simulink model "SMD_MSR_Sim_V1"  (R2019a)
settings: Solver=ode45  StartTime=0.0  StopTime=simtime  MaxStep=ts_max
values from neighbouring files (symbols this model uses):
  a_f = 1E-5*depl_fuel_temp_coef(depl_index)    [MSDR_parameters_V5.m]    (also in SMD_MSR_Para_V1.m)
  a_g = 1E-5*depl_grap_temp_coef(depl_index)    [MSDR_parameters_V5.m]    (also in SMD_MSR_Para_V1.m)
  beta = depl_beta(depl_index,:)    [MSDR_parameters_V5.m]    (also in SMD_MSR_Para_V1.m)
  beta_t = sum(beta)    [MSDR_parameters_V5.m]    (also in SMD_MSR_Para_V1.m)
  Block_UHE = 200000    [step_insertion_depl.m]
  DHRS_Power = P*(0.10)    (= 0.8)    [step_insertion_depl.m]
  DHRS_time = 200000    [step_insertion_depl.m]
  DHRS_TIME_K = 10    [MSDR_parameters_V5.m]    (also in SMD_MSR_Para_V1.m)
  Epsilon = 1E-3    (= 0.001)    [MSDR_parameters_V5.m]    (also in SMD_MSR_Para_V1.m)
  Fiss_factor = 2.464783802008740e-03    (= 0.00246478380201)    [MSDR_parameters_V5.m]    (also in SMD_MSR_Para_V1.m)
  gamma0 = 9.635981959409105e-01    (= 0.963598195941)    [MSDR_parameters_V5.m]    (also in SMD_MSR_Para_V1.m)
  gamma1 = 3.560674858154914e-02    (= 0.0356067485815)    [MSDR_parameters_V5.m]    (also in SMD_MSR_Para_V1.m)
  gamma2 = 7.950554775404400e-04    (= 0.00079505547754)    [MSDR_parameters_V5.m]    (also in SMD_MSR_Para_V1.m)
  gamma_I = 5.1135e-2    (= 0.051135)    [MSDR_parameters_V5.m]    (also in SMD_MSR_Para_V1.m)
  gamma_Xe = 1.1628e-2    (= 0.011628)    [MSDR_parameters_V5.m]    (also in SMD_MSR_Para_V1.m)
  hA_fg = [h_fg*A_fg/2, h_fg*A_fg/2]    [MSDR_parameters_V5.m]    (also in SMD_MSR_Para_V1.m = Psf_li*(0.02*9/5)/nn_f)
  hA_pn = (Psf_li*ha_p)/nn_s    [SMD_MSR_Para_V1.m]
  hA_rpn = (Psf_li*h_roverall*A_rad)/nn_rs    [SMD_MSR_Para_V1.m]
  hA_rsn = (Psf_li*h_roverall*A_rad)/nn_rs    [SMD_MSR_Para_V1.m]
  hA_sn = (Psf_li*ha_s)/nn_s    [SMD_MSR_Para_V1.m]
  I_0 = gamma_I*Sig_f_msdr*phi_0/lam_I    [MSDR_parameters_V5.m]    (also in SMD_MSR_Para_V1.m)
  k_1 = 0.5    [SMD_MSR_Para_V1.m]
  k_2 = 0.5    [SMD_MSR_Para_V1.m]
  k_f1 = k_f/nn_f    (= 0.465)    [SMD_MSR_Para_V1.m]
  k_f2 = k_f/nn_f    (= 0.465)    [SMD_MSR_Para_V1.m]
  k_g = 0.07    [SMD_MSR_Para_V1.m]
  K_pump = 1/5    (= 0.2)    [MSDR_parameters_V5.m]    (also in SMD_MSR_Para_V1.m = 10000000)
  Lam = depl_Lam(depl_index)    [MSDR_parameters_V5.m]    (also in SMD_MSR_Para_V1.m)
  lam = [0.0124, 0.0305, 0.111, 0.301, 1.14, 3.01]    [MSDR_parameters_V5.m]    (also in SMD_MSR_Para_V1.m = [1.240E-02, 3.05E-02, 1.11E-01, 3.01E-01, 1.140E+00, 3.014E+)
  lam_bubl = 2.0e-2    (= 0.02)    [MSDR_parameters_V5.m]    (also in SMD_MSR_Para_V1.m)
  lam_I = 2.875e-5    (= 2.875e-05)    [MSDR_parameters_V5.m]    (also in SMD_MSR_Para_V1.m)
  lam_Xe = 2.0916e-5    (= 2.0916e-05)    [MSDR_parameters_V5.m]    (also in SMD_MSR_Para_V1.m)
  lambda0 = 0.0945298    [MSDR_parameters_V5.m]    (also in SMD_MSR_Para_V1.m)
  lambda1 = 0.00441957    [MSDR_parameters_V5.m]    (also in SMD_MSR_Para_V1.m)
  lambda2 = 8.60979e-05    [MSDR_parameters_V5.m]    (also in SMD_MSR_Para_V1.m)
  m_f_t = total_mp_phx + core_fm    [MSDR_parameters_V5.m]    (also in SMD_MSR_Para_V1.m = W_f*(tau_l+tau_c))
  mcp_f1 = mn_f*scp_f    [SMD_MSR_Para_V1.m]
  mcp_f2 = mn_f*scp_f    [SMD_MSR_Para_V1.m]
  mcp_g1 = m_g*scp_g    [SMD_MSR_Para_V1.m]
  mcp_pn = mn_p*cp_p    [SMD_MSR_Para_V1.m]
  mcp_rpn = mn_rp*cp_rp    [SMD_MSR_Para_V1.m]
  mcp_rsn = mn_rs*scp_rs    [SMD_MSR_Para_V1.m]
  mcp_sn = mn_s*scp_s    [SMD_MSR_Para_V1.m]
  mcp_tn = m_tn*scp_t    [SMD_MSR_Para_V1.m]
  mn_f = (m_f/nn_f)    [SMD_MSR_Para_V1.m]
  mn_p = m_p/nn_p    [SMD_MSR_Para_V1.m]
  mn_pi_c_hx = W_f*tau_c_hx    (= 1783.7391)    [MSDR_parameters_V5.m]    (also in SMD_MSR_Para_V1.m = (W_f*tau_c_hx))
  mn_pi_hx_c = W_f*3*tau_hx_c + m_fm    (= 15330.1773)    [MSDR_parameters_V5.m]    (also in SMD_MSR_Para_V1.m = (W_f*tau_hx_c))
  mn_piDHRS = W_f*(0.1)    (= 498.948)    [MSDR_parameters_V5.m]    (also in SMD_MSR_Para_V1.m = (W_f*tau_DHRS))
  mn_piFP = (W_f*tau_FP)    [SMD_MSR_Para_V1.m]
  mn_rp = m_rp/nn_rp    [SMD_MSR_Para_V1.m]
  mn_rs = m_rs/nn_rs    [SMD_MSR_Para_V1.m]
  mn_s = m_s/nn_s    [SMD_MSR_Para_V1.m]
  n_frac0 = 1    [SMD_MSR_Para_V1.m]
  omega = 10.00000    (= 10)    [step_insertion_depl.m]
  P = 8    [step_insertion_depl.m]
  phi_0 = P/(3.04414e-17*1e6*Sig_f_msdr)    [MSDR_parameters_V5.m]    (also in SMD_MSR_Para_V1.m)
  Power_Bleed = P*(0.00)    [MSDR_parameters_V5.m]    (also in step_insertion_depl.m = 0)
  rho_f = 751.042    [MSDR_parameters_V5.m]    (also in SMD_MSR_Para_V1.m = 2146.47)
  rho_s = 1/vss    [MSDR_parameters_V5.m]    (also in SMD_MSR_Para_V1.m = 1922)
  rhoXe_0 = (-sig_Xe/Sig_a)*(gamma_I+gamma_Xe)*Sig_f_msdr*phi_0/(lam_Xe + sig_Xe*phi_0 + lam_bubl)    [MSDR_parameters_V5.m]    (also in SMD_MSR_Para_V1.m)
  rm_power = W_f*scp_f*deltaTf_DHRS    [SMD_MSR_Para_V1.m]
  scp_f = 1.9665E-3    (= 0.0019665)    [SMD_MSR_Para_V1.m]
  scp_s = 2.39E-3    (= 0.00239)    [SMD_MSR_Para_V1.m]
  Sig_f_msdr = U_den*U_sig    [MSDR_parameters_V5.m]    (also in SMD_MSR_Para_V1.m = 0.058501076601)
  sig_Xe = 2.66449e-18    [MSDR_parameters_V5.m]    (also in SMD_MSR_Para_V1.m)
  sin_mag = 0    [step_insertion_depl.m]
  slug_time = 8.46    [step_insertion_depl.m]
  T0_f1 = Tf_in + (T0_f2-Tf_in)/2    (= 644.745)    [SMD_MSR_Para_V1.m]
  T0_f2 = 6.5727E+02    (= 657.27)    [SMD_MSR_Para_V1.m]
  T0_g1 = T0_f1+(k_g*P_MSRE/hA_fg)    [SMD_MSR_Para_V1.m]
  T0_p1 = Tp_in - (Tp_in-T0_p4)/4    (= 651.0075)    [SMD_MSR_Para_V1.m]
  T0_p2 = Tp_in - 2*(Tp_in-T0_p4)/4    (= 644.745)    [SMD_MSR_Para_V1.m]
  T0_p3 = Tp_in - 3*(Tp_in-T0_p4)/4    (= 638.4825)    [SMD_MSR_Para_V1.m]
  T0_p4 = Tf_in    (= 632.22)    [SMD_MSR_Para_V1.m]
  T0_rp = Ts_in    (= 546.11)    [SMD_MSR_Para_V1.m]
  T0_rs = 148.9    [SMD_MSR_Para_V1.m]
  T0_s1 = Ts_in + (T0_s4-Ts_in)/nn_s    (= 554.43)    [SMD_MSR_Para_V1.m]
  T0_s2 = Ts_in + 2*(T0_s4-Ts_in)/nn_s    (= 562.75)    [SMD_MSR_Para_V1.m]
  T0_s3 = Ts_in + 3*(T0_s4-Ts_in)/nn_s    (= 571.07)    [SMD_MSR_Para_V1.m]
  T0_s4 = 5.7939E+02    (= 579.39)    [SMD_MSR_Para_V1.m]
  T0_t1 = 6.253671698113207E+02    (= 625.367169811)    [SMD_MSR_Para_V1.m]
  T0_t2 = 6.115222641509436e+02    (= 611.522264151)    [SMD_MSR_Para_V1.m]
  tau_c = core_fm/W_f    [MSDR_parameters_V5.m]    (also in SMD_MSR_Para_V1.m = 8.46)
  tau_c_DHRS = (tau_c_hx - tau_DHRS)/2    (= 1.385)    [SMD_MSR_Para_V1.m]
  tau_DHRS_hx = (tau_c_hx - tau_DHRS)/2    (= 1.385)    [SMD_MSR_Para_V1.m]
  tau_FP_c = (tau_hx_c - tau_FP)/2    (= 3.835)    [SMD_MSR_Para_V1.m]
  tau_hx_FP = (tau_hx_c - tau_FP)/2    (= 3.835)    [SMD_MSR_Para_V1.m]
  tau_hx_r = 4.71    [SMD_MSR_Para_V1.m]
  tau_l = pipe_fm/W_f    [MSDR_parameters_V5.m]    (also in SMD_MSR_Para_V1.m = 16.73)
  tau_r_hx = 8.24    [SMD_MSR_Para_V1.m]
  Trip_P_pump = 20000000    [step_insertion_depl.m]
  Trip_S_pump = 20000000    [step_insertion_depl.m]
  Trs_in = 37.78    [SMD_MSR_Para_V1.m]
  vdot_f = Psf_li*7.5708E-02    [SMD_MSR_Para_V1.m]
  vdot_f_fc_pc = 0.05    [MSDR_parameters_V5.m]    (also in SMD_MSR_Para_V1.m)
  vdot_s = Psf_li*5.36265E-02    [SMD_MSR_Para_V1.m]
  W_f = 4989.48    [MSDR_parameters_V5.m]    (also in SMD_MSR_Para_V1.m = vdot_f*rho_f)
  W_p = W_f    [SMD_MSR_Para_V1.m]
  W_rp = W_s    [SMD_MSR_Para_V1.m]
  W_rs = vdot_rs*rho_rs    [SMD_MSR_Para_V1.m]
  W_s = vdot_s*rho_s    [SMD_MSR_Para_V1.m]
  Xe_0 = (gamma_Xe*Sig_f_msdr*phi_0 + lam_I*I_0)/(lam_Xe + sig_Xe*phi_0 + lam_bubl)    [MSDR_parameters_V5.m]    (also in SMD_MSR_Para_V1.m)
  Xe_og = lam_bubl*Xe_0/(lam_Xe)    [MSDR_parameters_V5.m]    (also in SMD_MSR_Para_V1.m)
undefined symbols (not defined in the file or in its folder): C0, ln
settings Model: Creator=visura96  LastModifiedBy=visura
settings SolverCC: AlgebraicLoopSolver=LineSearch
settings DataIOCC: ReturnWorkspaceOutputs=off

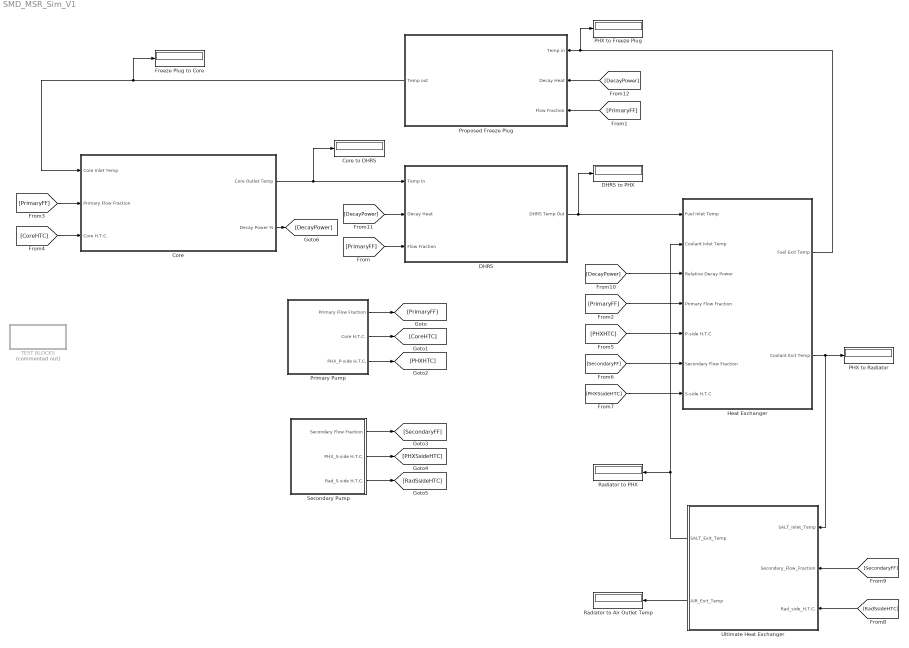
== system SMD_MSR_Sim_V1 ==
  " Heat Exchanger" : Subsystem
  Core : Subsystem
  Core to DHRS : Display
  "DHRS " : Subsystem
  DHRS to PHX : Display
  Freeze Plug to Core : Display
  PHX to Freeze Plug : Display
  PHX to Radiator : Display
  Primary Pump : Subsystem
  Proposed Freeze Plug : Subsystem
  Radiator to Air Outlet Temp : Display
  Radiator to PHX : Display
  Secondary Pump : Subsystem
  TEST BLOCKS : Subsystem  Commented=on
  Ultimate Heat Exchanger : Subsystem  Variant=on
  wires:
  Primary Pump/1(Primary Flow Fraction) -> [PrimaryFF]
  [PrimaryFF] -> Proposed Freeze Plug/3(Flow Fraction)
  [PrimaryFF] -> " Heat Exchanger"/4(Primary Flow Fraction)
  [PrimaryFF] -> Core/2(Primary Flow Fraction)
  Primary Pump/2(Core H.T.C.) -> [CoreHTC]
  [CoreHTC] -> Core/3(Core H.T.C.)
  Primary Pump/3(PHX_P-side H.T.C.) -> [PHXHTC]
  [PHXHTC] -> " Heat Exchanger"/5(P-side H.T.C)
  Secondary Pump/1(Secondary Flow Fraction) -> [SecondaryFF]
  Secondary Pump/2(PHX_S-side H.T.C.) -> [PHXSsideHTC]
  Secondary Pump/3(Rad_S-side H.T.C.) -> [RadSsideHTC]
  [SecondaryFF] -> " Heat Exchanger"/6(Secondary Flow Fraction)
  [PHXSsideHTC] -> " Heat Exchanger"/7(S-side H.T.C)
  [DecayPower] -> " Heat Exchanger"/3(Relative Decay Power)
  [DecayPower] -> Proposed Freeze Plug/2(Decay Heat)
  Core/1(Core Outlet Temp) -> Core to DHRS/1, "DHRS "/1("Temp In ")
  Core/2(Decay Power %) -> [DecayPower]
  [DecayPower] -> "DHRS "/2(Decay Heat)
  [PrimaryFF] -> "DHRS "/3(Flow Fraction)
  Proposed Freeze Plug/1(Temp out) -> Freeze Plug to Core/1, Core/1("Core Inlet Temp ")
  " Heat Exchanger"/2(Coolant Exit Temp) -> Ultimate Heat Exchanger/1(SALT_Inlet_Temp), PHX to Radiator/1
  "DHRS "/1("DHRS Temp Out ") -> " Heat Exchanger"/1(Fuel Inlet Temp), DHRS to PHX/1
  " Heat Exchanger"/1(Fuel Exit Temp) -> PHX to Freeze Plug/1, Proposed Freeze Plug/1("Temp in ")
  [RadSsideHTC] -> Ultimate Heat Exchanger/3(Rad_side_H.T.C.)
  [SecondaryFF] -> Ultimate Heat Exchanger/2(Secondary_Flow_Fraction)
  Ultimate Heat Exchanger/1(SALT_Exit_Temp) -> Radiator to PHX/1, " Heat Exchanger"/2(Coolant Inlet Temp)
  Ultimate Heat Exchanger/2(AIR_Exit_Temp) -> Radiator to Air Outlet Temp/1

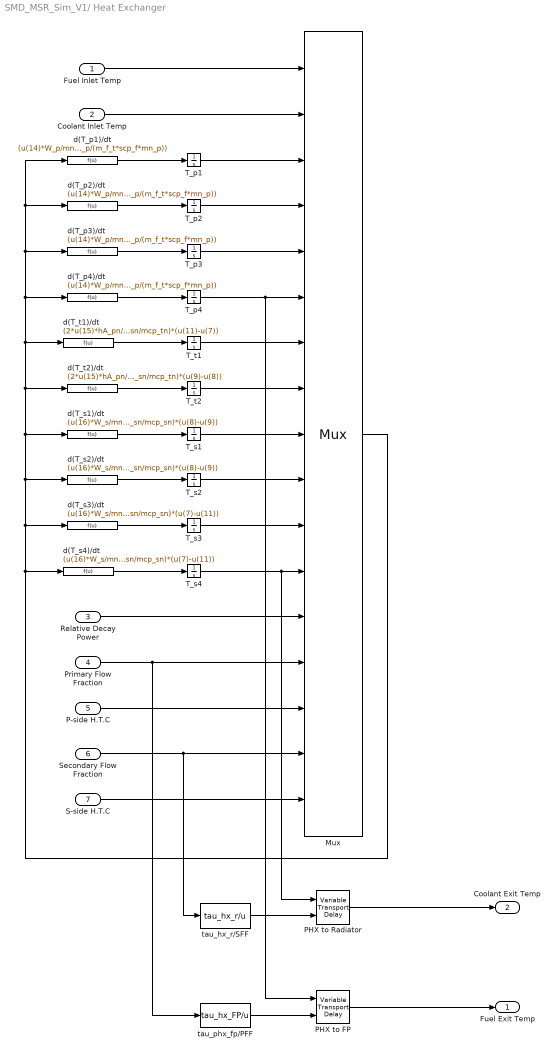
== system SMD_MSR_Sim_V1/ Heat Exchanger ==
  Fuel Inlet Temp : Inport
  Coolant Inlet Temp : Inport  Port=2
  Relative Decay Power : Inport  Port=3
  Primary Flow Fraction : Inport  Port=4
  P-side H.T.C : Inport  Port=5
  Secondary Flow Fraction : Inport  Port=6
  S-side H.T.C : Inport  Port=7
  Mux : Mux  Inputs=17
      settings: DisplayOption=signals
  PHX to FP : VariableTransportDelay  MaximumDelay=10000000000  InitialOutput=T0_p4
  PHX to Radiator : VariableTransportDelay  MaximumDelay=10000000000  InitialOutput=T0_s4
  T_p1 : Integrator  InitialCondition=T0_p1
  T_p2 : Integrator  InitialCondition=T0_p2
  "T_p3 " : Integrator  InitialCondition=T0_p3
  T_p4 : Integrator  InitialCondition=T0_p4
  T_s1 : Integrator  InitialCondition=T0_s1
  T_s2 : Integrator  InitialCondition=T0_s2
  T_s3 : Integrator  InitialCondition=T0_s3
  T_s4 : Integrator  InitialCondition=T0_s4
  T_t1 : Integrator  InitialCondition=T0_t1
  T_t2 : Integrator  InitialCondition=T0_t2
  d(T_p1)/dt : Fcn  Expr=(u(14)*W_p/mn_p)*(u(1)-u(3)) + (u(15)*hA_pn/mcp_pn)*(u(7)-u(3)) + (u(13)*P*mn_p/(m_f_t*scp_f*mn_p))
  d(T_p2)/dt : Fcn  Expr=(u(14)*W_p/mn_p)*(u(3)-u(4)) + (u(15)*hA_pn/mcp_pn)*(u(7)-u(3)) + (u(13)*P*mn_p/(m_f_t*scp_f*mn_p))
  d(T_p3)/dt : Fcn  Expr=(u(14)*W_p/mn_p)*(u(4)-u(5)) + (u(15)*hA_pn/mcp_pn)*(u(8)-u(5)) + (u(13)*P*mn_p/(m_f_t*scp_f*mn_p))
  d(T_p4)/dt : Fcn  Expr=(u(14)*W_p/mn_p)*(u(5)-u(6)) + (u(15)*hA_pn/mcp_pn)*(u(8)-u(5)) + (u(13)*P*mn_p/(m_f_t*scp_f*mn_p))
  d(T_s1)/dt : Fcn  Expr=(u(16)*W_s/mn_s)*(u(2)-u(9)) + (u(17)*hA_sn/mcp_sn)*(u(8)-u(9))
  d(T_s2)/dt : Fcn  Expr=(u(16)*W_s/mn_s)*(u(9)-u(10)) + (u(17)*hA_sn/mcp_sn)*(u(8)-u(9))
  d(T_s3)/dt : Fcn  Expr=(u(16)*W_s/mn_s)*(u(10)-u(11)) + (u(17)*hA_sn/mcp_sn)*(u(7)-u(11))
  d(T_s4)/dt : Fcn  Expr=(u(16)*W_s/mn_s)*(u(11)-u(12)) + (u(17)*hA_sn/mcp_sn)*(u(7)-u(11))
  d(T_t1)/dt : Fcn  Expr=(2*u(15)*hA_pn/mcp_tn)*(u(3)-u(7)) + (2*u(17)*hA_sn/mcp_tn)*(u(11)-u(7))
  d(T_t2)/dt : Fcn  Expr=(2*u(15)*hA_pn/mcp_tn)*(u(5)-u(8)) + (2*u(17)*hA_sn/mcp_tn)*(u(9)-u(8))
  tau_hx_r/SFF : Fcn  Expr=tau_hx_r/u
  tau_phx_fp/PFF : Fcn  Expr=tau_hx_FP/u
  Fuel Exit Temp : Outport
  Coolant Exit Temp : Outport  Port=2
  wires:
  Fuel Inlet Temp/1 -> Mux/1
  Coolant Inlet Temp/1 -> Mux/2
  d(T_p1)/dt/1 -> T_p1/1
  d(T_p2)/dt/1 -> T_p2/1
  d(T_p3)/dt/1 -> "T_p3 "/1
  d(T_p4)/dt/1 -> T_p4/1
  d(T_t1)/dt/1 -> T_t1/1
  d(T_t2)/dt/1 -> T_t2/1
  d(T_s1)/dt/1 -> T_s1/1
  d(T_s2)/dt/1 -> T_s2/1
  T_p2/1 -> Mux/4
  T_p1/1 -> Mux/3
  d(T_s3)/dt/1 -> T_s3/1
  d(T_s4)/dt/1 -> T_s4/1
  Mux/1 -> d(T_s4)/dt/1, d(T_s3)/dt/1, d(T_s2)/dt/1, d(T_s1)/dt/1, d(T_t2)/dt/1, d(T_t1)/dt/1, d(T_p4)/dt/1, d(T_p3)/dt/1, d(T_p2)/dt/1, d(T_p1)/dt/1
  "T_p3 "/1 -> Mux/5
  T_p4/1 -> PHX to FP/1, Mux/6
  T_t1/1 -> Mux/7
  T_s4/1 -> PHX to Radiator/1, Mux/12
  T_s3/1 -> Mux/11
  T_s2/1 -> Mux/10
  T_t2/1 -> Mux/8
  Relative Decay Power/1 -> Mux/13
  Primary Flow Fraction/1 -> tau_phx_fp/PFF/1, Mux/14
  P-side H.T.C/1 -> Mux/15
  Secondary Flow Fraction/1 -> tau_hx_r/SFF/1, Mux/16
  S-side H.T.C/1 -> Mux/17
  tau_hx_r/SFF/1 -> PHX to Radiator/2
  PHX to Radiator/1 -> Coolant Exit Temp/1
  T_s1/1 -> Mux/9
  PHX to FP/1 -> Fuel Exit Temp/1
  tau_phx_fp/PFF/1 -> PHX to FP/2

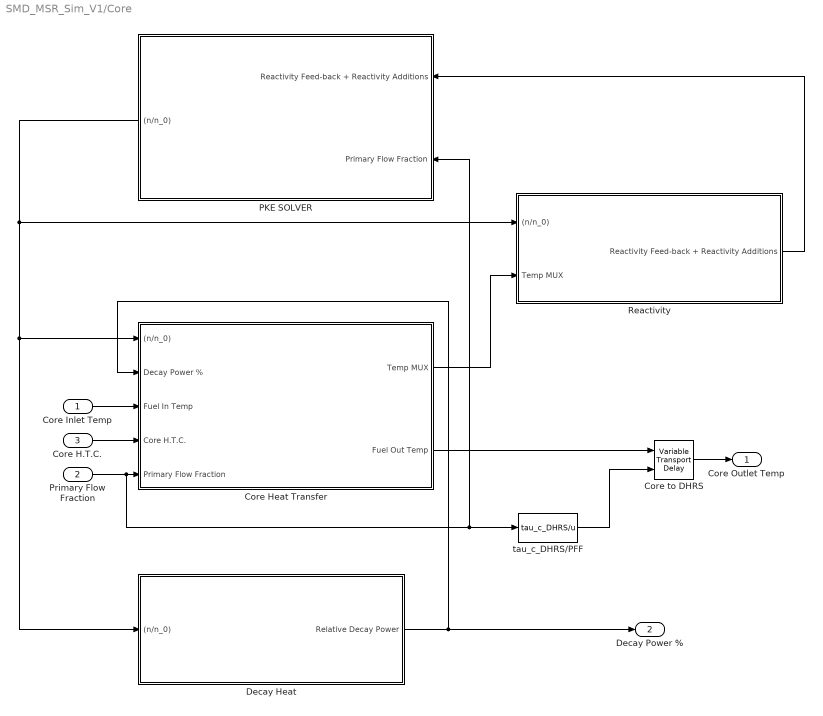
== system SMD_MSR_Sim_V1/Core ==
  "Core Inlet Temp " : Inport
  Primary Flow Fraction : Inport  Port=2
  Core H.T.C. : Inport  Port=3
  Core Heat Transfer : Subsystem
  Core to DHRS : VariableTransportDelay  MaximumDelay=10000000000  InitialOutput=T0_f2
  Decay Heat : Subsystem
  PKE SOLVER : Subsystem
  "Reactivity " : Subsystem
  tau_c_DHRS/PFF : Fcn  Expr=tau_c_DHRS/u
  Core Outlet Temp : Outport
  Decay Power % : Outport  Port=2
  wires:
  "Core Inlet Temp "/1 -> Core Heat Transfer/3(Fuel In Temp)
  Primary Flow Fraction/1 -> tau_c_DHRS/PFF/1, PKE SOLVER/2(Primary Flow Fraction), Core Heat Transfer/5(Primary Flow Fraction)
  Core H.T.C./1 -> Core Heat Transfer/4(Core H.T.C.)
  Core Heat Transfer/1(Temp MUX) -> "Reactivity "/2(Temp MUX)
  Decay Heat/1("Relative Decay Power ") -> Core Heat Transfer/2(Decay Power %), Decay Power %/1
  "Reactivity "/1(Reactivity Feed-back + Reactivity Additions) -> PKE SOLVER/1(Reactivity Feed-back + Reactivity Additions)
  PKE SOLVER/1((n/n_0)) -> Core Heat Transfer/1("(n/n_0) "), Decay Heat/1((n/n_0)), "Reactivity "/1((n/n_0))
  Core Heat Transfer/2(Fuel Out Temp) -> Core to DHRS/1
  Core to DHRS/1 -> Core Outlet Temp/1
  tau_c_DHRS/PFF/1 -> Core to DHRS/2

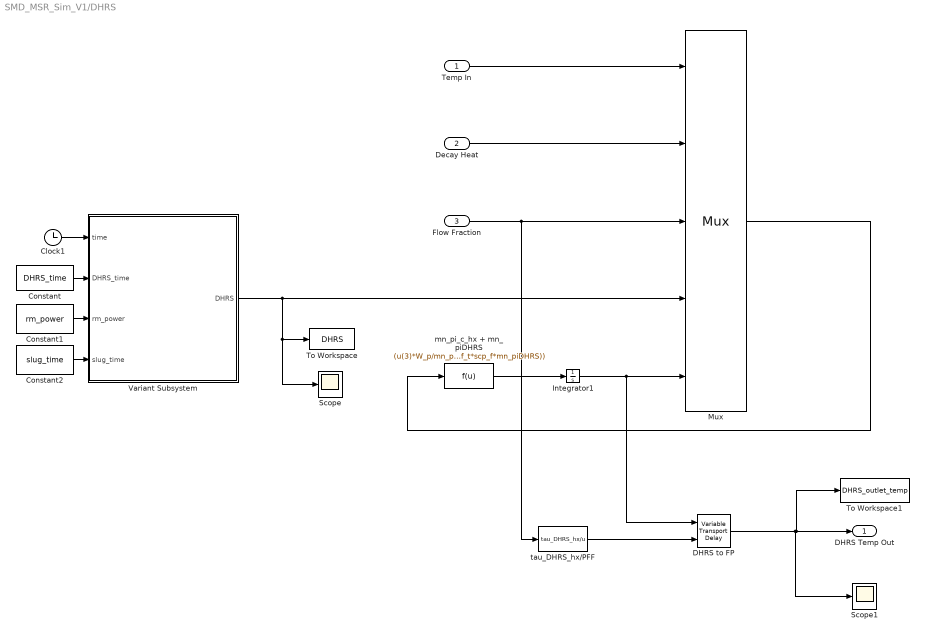
== system SMD_MSR_Sim_V1/DHRS  ==
  "Temp In " : Inport
  Decay Heat : Inport  Port=2
  Flow Fraction : Inport  Port=3
  Clock1 : Clock
  Constant : Constant  Value=DHRS_time
  Constant1 : Constant  Value=rm_power
  Constant2 : Constant  Value=slug_time
  DHRS to FP : VariableTransportDelay  MaximumDelay=10000000000  InitialOutput=T0_p1
  Integrator1 : Integrator  InitialCondition=T0_p1
  Mux : Mux  Inputs=5
      settings: DisplayOption=signals
  Scope : Scope
  Scope1 : Scope
  To Workspace : ToWorkspace  VariableName=DHRS  SaveFormat=Timeseries  SampleTime=-1
  To Workspace1 : ToWorkspace  VariableName=DHRS_outlet_temp  SampleTime=-1
  Variant Subsystem : Subsystem  Variant=on
  mn_pi_c_hx + mn_piDHRS : Fcn  Expr="(u(3)*W_p/mn_piDHRS)*(u(1) - u(5)) - (u(4)/(mn_piDHRS*scp_f))  + (u(2)*P*mn_pi_c_hx/(m_f_t*scp_f*mn_piDHRS))"
  tau_DHRS_hx/PFF : Fcn  Expr=tau_DHRS_hx/u
  "DHRS Temp Out " : Outport
  wires:
  Mux/1 -> mn_pi_c_hx + mn_piDHRS/1
  Flow Fraction/1 -> Mux/3, tau_DHRS_hx/PFF/1
  mn_pi_c_hx + mn_piDHRS/1 -> Integrator1/1
  DHRS to FP/1 -> Scope1/1, To Workspace1/1, "DHRS Temp Out "/1
  tau_DHRS_hx/PFF/1 -> DHRS to FP/2
  Integrator1/1 -> Mux/5, DHRS to FP/1
  Variant Subsystem/1(DHRS) -> To Workspace/1, Scope/1, Mux/4
  Clock1/1 -> Variant Subsystem/1(time)
  Constant/1 -> Variant Subsystem/2(DHRS_time)
  Constant1/1 -> Variant Subsystem/3(rm_power)
  Constant2/1 -> Variant Subsystem/4(slug_time)
  "Temp In "/1 -> Mux/1
  Decay Heat/1 -> Mux/2

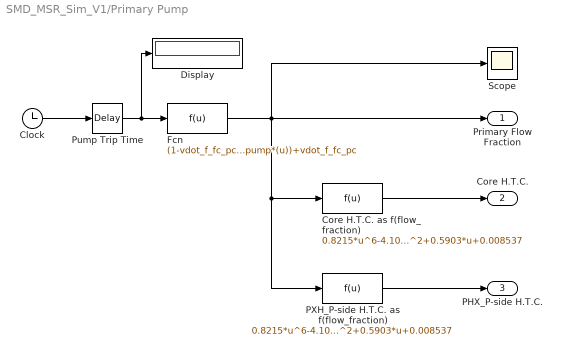
== system SMD_MSR_Sim_V1/Primary Pump ==
  Clock : Clock
  Core H.T.C. as f(flow_fraction) : Fcn  Expr=0.8215*u^6-4.108*u^5+7.848*u^4-7.165*u^3+3.004*u^2+0.5903*u+0.008537
  Display : Display
  Fcn : Fcn  Expr=(1-vdot_f_fc_pc)*exp(-K_pump*(u))+vdot_f_fc_pc
  PXH_P-side H.T.C. as f(flow_fraction) : Fcn  Expr=0.8215*u^6-4.108*u^5+7.848*u^4-7.165*u^3+3.004*u^2+0.5903*u+0.008537
  Pump Trip Time : TransportDelay  DelayTime=Trip_P_pump  BufferSize=4096
  Scope : Scope
  Primary Flow Fraction : Outport
  Core H.T.C. : Outport  Port=2
  PHX_P-side H.T.C. : Outport  Port=3
  wires:
  Fcn/1 -> Primary Flow Fraction/1, Scope/1, PXH_P-side H.T.C. as f(flow_fraction)/1, Core H.T.C. as f(flow_fraction)/1
  Clock/1 -> Pump Trip Time/1
  Pump Trip Time/1 -> Display/1, Fcn/1
  Core H.T.C. as f(flow_fraction)/1 -> Core H.T.C./1
  PXH_P-side H.T.C. as f(flow_fraction)/1 -> PHX_P-side H.T.C./1

== system SMD_MSR_Sim_V1/Proposed Freeze Plug ==
  "Temp in " : Inport
  Decay Heat : Inport  Port=2
  Flow Fraction : Inport  Port=3
  FP to Core : VariableTransportDelay  MaximumDelay=10000000000  InitialOutput=T0_p4
  Mux : Mux
      settings: DisplayOption=signals
  "Pipe Node 1 " : Fcn  Expr=(u(3)*W_p/mn_piFP)*(u(1)-u(4)) + (u(2)*P*mn_pi_hx_c/(m_f_t*scp_f*mn_piFP))
  T_p4 : Integrator  InitialCondition=T0_p4
  tau_fp_c/PFF : Fcn  Expr=tau_FP_c/u
  Temp out : Outport
  wires:
  "Temp in "/1 -> Mux/1
  "Pipe Node 1 "/1 -> T_p4/1
  Decay Heat/1 -> Mux/2
  Flow Fraction/1 -> Mux/3, tau_fp_c/PFF/1
  Mux/1 -> "Pipe Node 1 "/1
  FP to Core/1 -> Temp out/1
  T_p4/1 -> FP to Core/1, Mux/4
  tau_fp_c/PFF/1 -> FP to Core/2

== system SMD_MSR_Sim_V1/Secondary Pump ==
  Clock1 : Clock
  Fcn : Fcn  Expr=(1-vdot_f_fc_pc)*exp(-K_pump*(u))+vdot_f_fc_pc
  PHX_S-side H.T.C. as f(flow_fraction) : Fcn  Expr=0.8215*u^6-4.108*u^5+7.848*u^4-7.165*u^3+3.004*u^2+0.5903*u+0.008537
  Pump Trip Time : TransportDelay  DelayTime=Trip_S_pump  BufferSize=4096
  Radiator_S-side H.T.C. as f(flow_fraction) : Fcn  Expr=0.8215*u^6-4.108*u^5+7.848*u^4-7.165*u^3+3.004*u^2+0.5903*u+0.008537
  Scope : Scope
  Secondary Flow Fraction : Outport
  PHX_S-side H.T.C. : Outport  Port=2
  Rad_S-side H.T.C. : Outport  Port=3
  wires:
  Fcn/1 -> Radiator_S-side H.T.C. as f(flow_fraction)/1, PHX_S-side H.T.C. as f(flow_fraction)/1, Secondary Flow Fraction/1, Scope/1
  Clock1/1 -> Pump Trip Time/1
  Pump Trip Time/1 -> Fcn/1
  PHX_S-side H.T.C. as f(flow_fraction)/1 -> PHX_S-side H.T.C./1
  Radiator_S-side H.T.C. as f(flow_fraction)/1 -> Rad_S-side H.T.C./1

== system SMD_MSR_Sim_V1/TEST BLOCKS ==
  Primary loop constant heat production : Subsystem  Commented=through
  Primary loop constant heat removal : Subsystem  Commented=through
  Secondaary loop constant heat production : Subsystem  Commented=through
  Secondary loop constant heat removal : Subsystem  Commented=through

== system SMD_MSR_Sim_V1/Ultimate Heat Exchanger ==
  SALT_Inlet_Temp : Inport
  Secondary_Flow_Fraction : Inport  Port=2
  Rad_side_H.T.C. : Inport  Port=3
  Radiator : Subsystem  VariantControl=Radiator
  UHX : Subsystem  VariantControl=UHX
  SALT_Exit_Temp : Outport
  AIR_Exit_Temp : Outport  Port=2

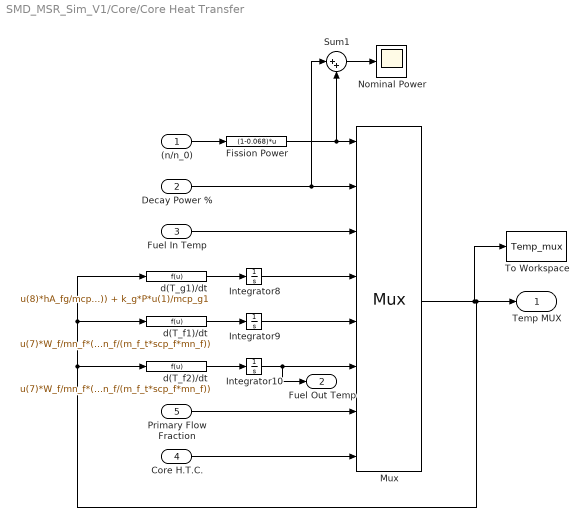
== system SMD_MSR_Sim_V1/Core/Core Heat Transfer ==
  "(n/n_0) " : Inport
  Decay Power % : Inport  Port=2
  Fuel In Temp : Inport  Port=3
  Core H.T.C. : Inport  Port=4
  Primary Flow Fraction : Inport  Port=5
  Fission Power : Fcn  Expr=(1-0.068)*u
  Integrator10 : Integrator  InitialCondition=T0_f2
  Integrator8 : Integrator  InitialCondition=T0_g1
  Integrator9 : Integrator  InitialCondition=T0_f1
  Mux : Mux  Inputs=8
      settings: DisplayOption=signals
  Nominal Power : Scope
  Sum1 : Sum  Inputs=|++
  To Workspace : ToWorkspace  VariableName=Temp_mux  SampleTime=-1
  d(T_f1)/dt : Fcn  Expr=u(7)*W_f/mn_f*(u(3) - u(5)) + (k_f1*P*u(1)/mcp_f1) + (u(8)*hA_fg*k_1*(u(4) - u(5))/mcp_f1) + (u(2)*P*mn_f/(m_f_t*scp_f*mn_f))
  d(T_f2)/dt : Fcn  Expr="u(7)*W_f/mn_f*(u(5) - u(6)) + (k_f2*P*u(1)/mcp_f2) + (u(8)*hA_fg*k_2*(u(4) - u(5))/mcp_f2)  + (u(2)*P*mn_f/(m_f_t*scp_f*mn_f))"
  d(T_g1)/dt : Fcn  Expr=u(8)*hA_fg/mcp_g1*(u(5) - u(4)) + k_g*P*u(1)/mcp_g1
  Temp MUX : Outport
  Fuel Out Temp : Outport  Port=2
  wires:
  d(T_g1)/dt/1 -> Integrator8/1
  d(T_f1)/dt/1 -> Integrator9/1
  d(T_f2)/dt/1 -> Integrator10/1
  Integrator10/1 -> Fuel Out Temp/1, Mux/6
  Integrator9/1 -> Mux/5
  Integrator8/1 -> Mux/4
  Mux/1 -> To Workspace/1, d(T_g1)/dt/1, d(T_f1)/dt/1, d(T_f2)/dt/1, Temp MUX/1
  Decay Power %/1 -> Sum1/1, Mux/2
  Fuel In Temp/1 -> Mux/3
  "(n/n_0) "/1 -> Fission Power/1
  Fission Power/1 -> Mux/1, Sum1/2
  Sum1/1 -> Nominal Power/1
  Primary Flow Fraction/1 -> Mux/7
  Core H.T.C./1 -> Mux/8

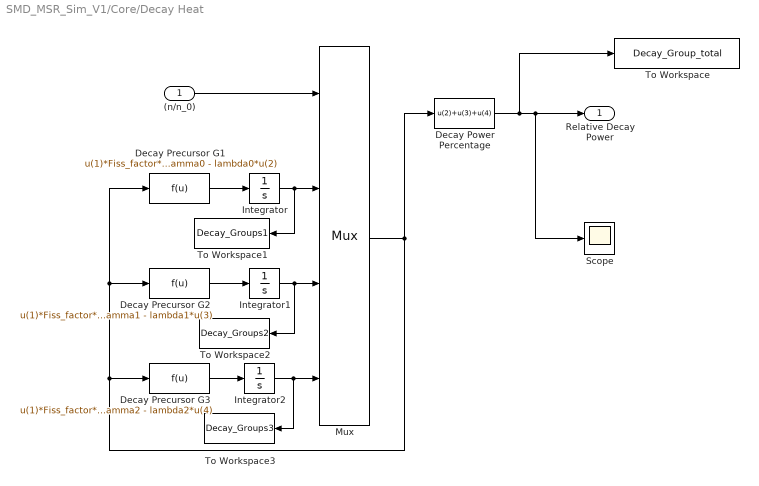
== system SMD_MSR_Sim_V1/Core/Decay Heat ==
  (n/n_0) : Inport
  Decay Power Percentage : Fcn  Expr=u(2)+u(3)+u(4)
  Decay Precursor G1 : Fcn  Expr=u(1)*Fiss_factor*gamma0 - lambda0*u(2)
  Decay Precursor G2 : Fcn  Expr=u(1)*Fiss_factor*gamma1 - lambda1*u(3)
  Decay Precursor G3 : Fcn  Expr=u(1)*Fiss_factor*gamma2 - lambda2*u(4)
  Integrator : Integrator  InitialCondition=0.025125
  Integrator1 : Integrator  InitialCondition=0.0198578
  Integrator2 : Integrator  InitialCondition=0.0227606
  Mux : Mux
      settings: DisplayOption=signals
  Scope : Scope
  To Workspace : ToWorkspace  VariableName=Decay_Group_total  SampleTime=-1
  To Workspace1 : ToWorkspace  VariableName=Decay_Groups1  SampleTime=-1
  To Workspace2 : ToWorkspace  VariableName=Decay_Groups2  SampleTime=-1
  To Workspace3 : ToWorkspace  VariableName=Decay_Groups3  SampleTime=-1
  "Relative Decay Power " : Outport
  wires:
  Decay Power Percentage/1 -> "Relative Decay Power "/1, Scope/1, To Workspace/1
  Decay Precursor G1/1 -> Integrator/1
  Decay Precursor G2/1 -> Integrator1/1
  Decay Precursor G3/1 -> Integrator2/1
  Mux/1 -> Decay Precursor G3/1, Decay Precursor G2/1, Decay Precursor G1/1, Decay Power Percentage/1
  Integrator/1 -> Mux/2, To Workspace1/1
  Integrator1/1 -> Mux/3, To Workspace2/1
  Integrator2/1 -> Mux/4, To Workspace3/1
  (n/n_0)/1 -> Mux/1

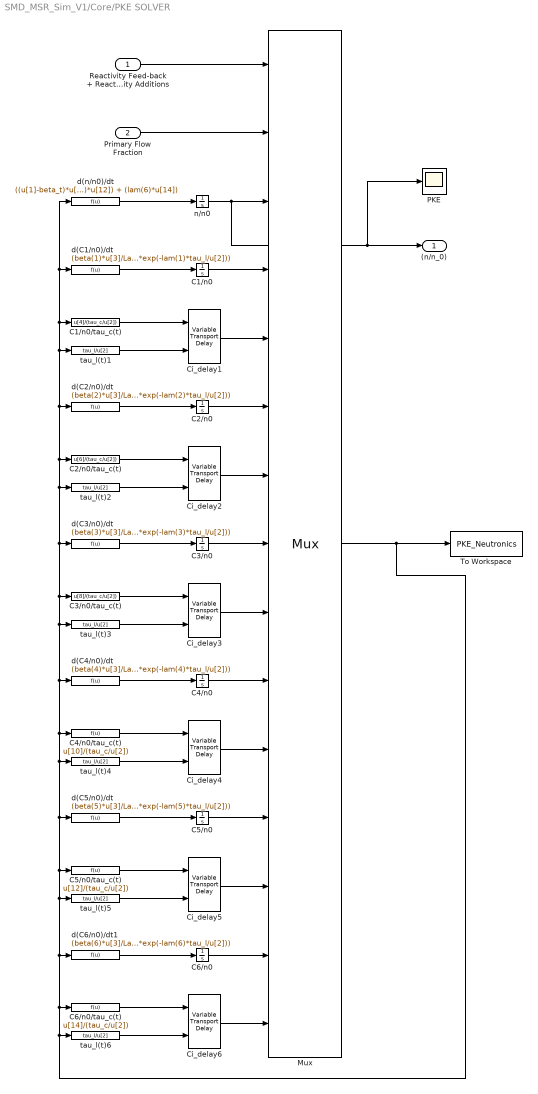
== system SMD_MSR_Sim_V1/Core/PKE SOLVER ==
  Reactivity Feed-back + Reactivity Additions : Inport
  Primary Flow Fraction : Inport  Port=2
  C1/n0 : Integrator  InitialCondition=C0(1)
  C1/n0/tau_c(t) : Fcn  Expr=u[4]/(tau_c/u[2])
  C2/n0 : Integrator  InitialCondition=C0(2)
  C2/n0/tau_c(t) : Fcn  Expr=u[6]/(tau_c/u[2])
  C3/n0 : Integrator  InitialCondition=C0(3)
  C3/n0/tau_c(t) : Fcn  Expr=u[8]/(tau_c/u[2])
  C4/n0 : Integrator  InitialCondition=C0(4)
  C4/n0/tau_c(t) : Fcn  Expr=u[10]/(tau_c/u[2])
  C5/n0 : Integrator  InitialCondition=C0(5)
  C5/n0/tau_c(t) : Fcn  Expr=u[12]/(tau_c/u[2])
  C6/n0 : Integrator  InitialCondition=C0(6)
  C6/n0/tau_c(t) : Fcn  Expr=u[14]/(tau_c/u[2])
  Ci_delay1 : VariableTransportDelay  MaximumDelay=10000000000  InitialOutput=C0(1)/tau_c
  Ci_delay2 : VariableTransportDelay  MaximumDelay=10000000000  InitialOutput=C0(2)/tau_c
  Ci_delay3 : VariableTransportDelay  MaximumDelay=10000000000  InitialOutput=C0(3)/tau_c
  Ci_delay4 : VariableTransportDelay  MaximumDelay=10000000000000  InitialOutput=C0(4)/tau_c
  Ci_delay5 : VariableTransportDelay  MaximumDelay=10000000000  InitialOutput=C0(5)/tau_c
  Ci_delay6 : VariableTransportDelay  MaximumDelay=10000000000000  InitialOutput=C0(6)/tau_c
  Mux : Mux  Inputs=15
      settings: DisplayOption=signals
  PKE : Scope
  To Workspace : ToWorkspace  VariableName=PKE_Neutronics  SampleTime=-1
  d(C1/n0)/dt : Fcn  Expr=(beta(1)*u[3]/Lam) - (lam(1)*u[4]) - (u[4]/(tau_c/u[2])) + (u[5]*exp(-lam(1)*tau_l/u[2]))
  d(C2/n0)/dt : Fcn  Expr=(beta(2)*u[3]/Lam) - (lam(2)*u[6]) - (u[6]/(tau_c/u[2])) + (u[7]*exp(-lam(2)*tau_l/u[2]))
  d(C3/n0)/dt : Fcn  Expr=(beta(3)*u[3]/Lam) - (lam(3)*u[8]) - (u[8]/(tau_c/u[2])) + (u[9]*exp(-lam(3)*tau_l/u[2]))
  d(C4/n0)/dt : Fcn  Expr=(beta(4)*u[3]/Lam) - (lam(4)*u[10]) - (u[10]/(tau_c/u[2])) + (u[11]*exp(-lam(4)*tau_l/u[2]))
  d(C5/n0)/dt : Fcn  Expr=(beta(5)*u[3]/Lam) - (lam(5)*u[12]) - (u[12]/(tau_c/u[2])) + (u[13]*exp(-lam(5)*tau_l/u[2]))
  d(C6/n0)/dt1 : Fcn  Expr=(beta(6)*u[3]/Lam) - (lam(6)*u[14]) - (u[14]/(tau_c/u[2])) + (u[14]*exp(-lam(6)*tau_l/u[2]))
  d(n/n0)/dt : Fcn  Expr=((u[1]-beta_t)*u[3]/Lam) + (lam(1)*u[4]) + (lam(2)*u[6]) + (lam(3)*u[8]) + (lam(4)*u[10]) + (lam(5)*u[12]) + (lam(6)*u[14])
  n/n0 : Integrator  InitialCondition=n_frac0
  tau_l(t){1..6} (6 alike) : Fcn  Expr=tau_l/u[2]
  (n/n_0) : Outport
  wires:
  C1/n0/tau_c(t)/1 -> Ci_delay1/1
  d(n/n0)/dt/1 -> n/n0/1
  d(C1/n0)/dt/1 -> C1/n0/1
  Reactivity Feed-back + Reactivity Additions/1 -> Mux/1
  n/n0/1 -> PKE/1, (n/n_0)/1, Mux/3
  Primary Flow Fraction/1 -> Mux/2
  C1/n0/1 -> Mux/4
  Ci_delay1/1 -> Mux/5
  tau_l(t)1/1 -> Ci_delay1/2
  C2/n0/tau_c(t)/1 -> Ci_delay2/1
  d(C2/n0)/dt/1 -> C2/n0/1
  tau_l(t)2/1 -> Ci_delay2/2
  Ci_delay2/1 -> Mux/7
  C2/n0/1 -> Mux/6
  C3/n0/1 -> Mux/8
  d(C3/n0)/dt/1 -> C3/n0/1
  tau_l(t)3/1 -> Ci_delay3/2
  Ci_delay3/1 -> Mux/9
  C3/n0/tau_c(t)/1 -> Ci_delay3/1
  C4/n0/1 -> Mux/10
  C4/n0/tau_c(t)/1 -> Ci_delay4/1
  tau_l(t)4/1 -> Ci_delay4/2
  d(C4/n0)/dt/1 -> C4/n0/1
  Ci_delay4/1 -> Mux/11
  C5/n0/tau_c(t)/1 -> Ci_delay5/1
  d(C5/n0)/dt/1 -> C5/n0/1
  tau_l(t)5/1 -> Ci_delay5/2
  C5/n0/1 -> Mux/12
  Ci_delay5/1 -> Mux/13
  C6/n0/1 -> Mux/14
  tau_l(t)6/1 -> Ci_delay6/2
  d(C6/n0)/dt1/1 -> C6/n0/1
  C6/n0/tau_c(t)/1 -> Ci_delay6/1
  Ci_delay6/1 -> Mux/15
  Mux/1 -> To Workspace/1, tau_l(t)4/1, d(n/n0)/dt/1, d(C1/n0)/dt/1, C1/n0/tau_c(t)/1, tau_l(t)1/1, d(C2/n0)/dt/1, C2/n0/tau_c(t)/1, tau_l(t)2/1, d(C3/n0)/dt/1, C3/n0/tau_c(t)/1, tau_l(t)3/1, d(C4/n0)/dt/1, C4/n0/tau_c(t)/1, d(C5/n0)/dt/1, C5/n0/tau_c(t)/1, tau_l(t)5/1, d(C6/n0)/dt1/1, C6/n0/tau_c(t)/1, tau_l(t)6/1

== system SMD_MSR_Sim_V1/Core/Reactivity  ==
  (n/n_0) : Inport
  Temp MUX : Inport  Port=2
  Temp + Reactity Insertions : Subsystem
  Xe Reactivity : Subsystem  Commented=on
  Reactivity Feed-back + Reactivity Additions : Outport
  wires:
  (n/n_0)/1 -> Xe Reactivity/1(n0)
  Temp MUX/1 -> Temp + Reactity Insertions/1("Temp MUX ")
  Temp + Reactity Insertions/1(Reactivity Feedback) -> Reactivity Feed-back + Reactivity Additions/1
  Xe Reactivity/1(drho_Xe) -> Temp + Reactity Insertions/2(Xe Reactivity)

== system SMD_MSR_Sim_V1/DHRS /Variant Subsystem ==
  time : Inport
  DHRS_time : Inport  Port=2
  rm_power : Inport  Port=3
  slug_time : Inport  Port=4
  Broken_DHRS : MATLAB Function  TreatAsAtomicUnit=on  VariantControl=Broken_DHRS
  Normal_DHRS : Subsystem  VariantControl=Normal_DHRS
  DHRS : Outport

== system SMD_MSR_Sim_V1/TEST BLOCKS/Primary loop constant heat production ==
  In1 : Inport
  Fcn : Fcn  Expr=u(1) + P/(vdot_f*rho_f*scp_f)
  Mux : Mux  Inputs=2
  Out1 : Outport
  wires:
  In1/1 -> Mux/1
  Fcn/1 -> Out1/1, Mux/2
  Mux/1 -> Fcn/1

== system SMD_MSR_Sim_V1/TEST BLOCKS/Primary loop constant heat removal ==
  In1 : Inport
  Fcn : Fcn  Expr=u(1) - P/(vdot_f*rho_f*scp_f)
  Mux : Mux  Inputs=2
  Out1 : Outport
  wires:
  In1/1 -> Mux/1
  Fcn/1 -> Out1/1, Mux/2
  Mux/1 -> Fcn/1

== system SMD_MSR_Sim_V1/TEST BLOCKS/Secondaary loop constant heat production ==
  In1 : Inport
  Fcn : Fcn  Expr=u(1) + P/(vdot_s*rho_s*scp_s)
  Mux : Mux  Inputs=2
  Out1 : Outport
  wires:
  In1/1 -> Mux/1
  Fcn/1 -> Out1/1, Mux/2
  Mux/1 -> Fcn/1

== system SMD_MSR_Sim_V1/TEST BLOCKS/Secondary loop constant heat removal ==
  In1 : Inport
  Fcn : Fcn  Expr=u(1) - P/(vdot_s*rho_s*scp_s)
  Mux : Mux  Inputs=2
  Out1 : Outport
  wires:
  In1/1 -> Mux/1
  Fcn/1 -> Out1/1, Mux/2
  Mux/1 -> Fcn/1

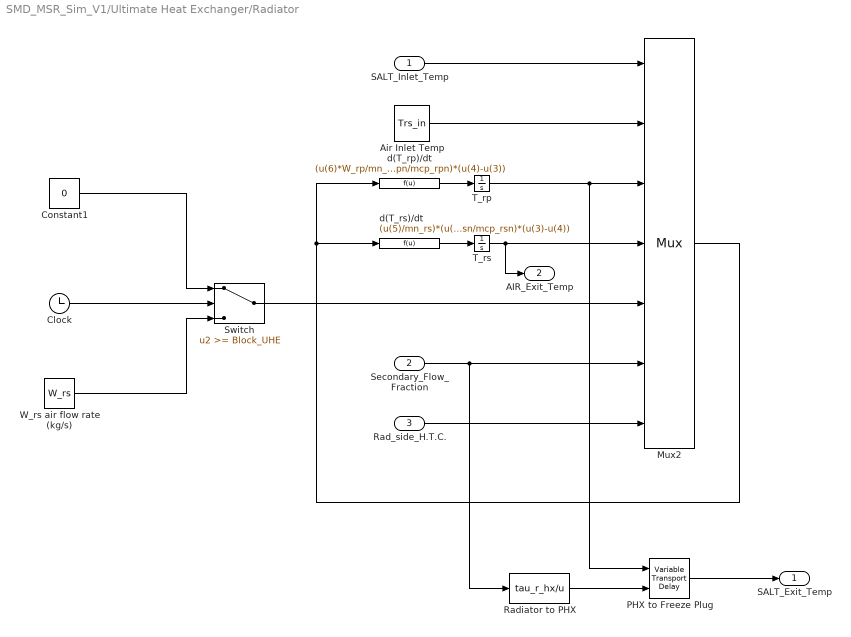
== system SMD_MSR_Sim_V1/Ultimate Heat Exchanger/Radiator ==
  SALT_Inlet_Temp : Inport
  Secondary_Flow_Fraction : Inport  Port=2
  Rad_side_H.T.C. : Inport  Port=3
  Air Inlet Temp : Constant  Value=Trs_in
  Clock : Clock
  Constant1 : Constant  Value=0
  Mux2 : Mux  Inputs=7
      settings: DisplayOption=signals
  PHX to Freeze Plug : VariableTransportDelay  MaximumDelay=10000000000  InitialOutput=T0_rp
  Radiator to PHX : Fcn  Expr=tau_r_hx/u
  Switch : Switch  Threshold=Block_UHE
  T_rp : Integrator  InitialCondition=T0_rp
  T_rs : Integrator  InitialCondition=T0_rs
  W_rs air flow rate (kg/s) : Constant  Value=W_rs
  d(T_rp)/dt : Fcn  Expr=(u(6)*W_rp/mn_rp)*(u(1)-u(3)) + (u(7)*hA_rpn/mcp_rpn)*(u(4)-u(3))
  d(T_rs)/dt : Fcn  Expr=(u(5)/mn_rs)*(u(2)-u(4)) + (u(7)*hA_rsn/mcp_rsn)*(u(3)-u(4))
  SALT_Exit_Temp : Outport
  AIR_Exit_Temp : Outport  Port=2
  wires:
  SALT_Inlet_Temp/1 -> Mux2/1
  d(T_rp)/dt/1 -> T_rp/1
  T_rp/1 -> PHX to Freeze Plug/1, Mux2/3
  d(T_rs)/dt/1 -> T_rs/1
  T_rs/1 -> AIR_Exit_Temp/1, Mux2/4
  Mux2/1 -> d(T_rs)/dt/1, d(T_rp)/dt/1
  Clock/1 -> Switch/2
  Constant1/1 -> Switch/1
  W_rs air flow rate (kg/s)/1 -> Switch/3
  Secondary_Flow_Fraction/1 -> Radiator to PHX/1, Mux2/6
  Rad_side_H.T.C./1 -> Mux2/7
  Radiator to PHX/1 -> PHX to Freeze Plug/2
  PHX to Freeze Plug/1 -> SALT_Exit_Temp/1
  Switch/1 -> Mux2/5
  Air Inlet Temp/1 -> Mux2/2

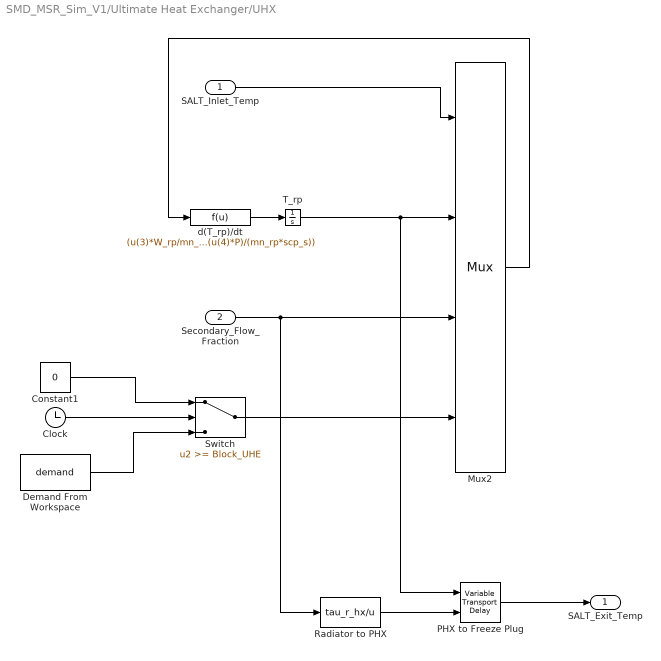
== system SMD_MSR_Sim_V1/Ultimate Heat Exchanger/UHX ==
  SALT_Inlet_Temp : Inport
  Secondary_Flow_Fraction : Inport  Port=2
  Clock : Clock
  Constant1 : Constant  Value=0
  Demand From Workspace : FromWorkspace  VariableName=demand  SampleTime=1  Interpolate=off  OutputAfterFinalValue=Holding final value
  Mux2 : Mux
      settings: DisplayOption=signals
  PHX to Freeze Plug : VariableTransportDelay  MaximumDelay=10000000000  InitialOutput=T0_rp
  Radiator to PHX : Fcn  Expr=tau_r_hx/u
  Switch : Switch  Threshold=Block_UHE
  T_rp : Integrator  InitialCondition=T0_rp
  d(T_rp)/dt : Fcn  Expr=(u(3)*W_rp/mn_rp)*(u(1)-u(2)) - ((u(4)*P)/(mn_rp*scp_s))
  SALT_Exit_Temp : Outport
  wires:
  SALT_Inlet_Temp/1 -> Mux2/1
  d(T_rp)/dt/1 -> T_rp/1
  T_rp/1 -> Mux2/2, PHX to Freeze Plug/1
  Mux2/1 -> d(T_rp)/dt/1
  Secondary_Flow_Fraction/1 -> Radiator to PHX/1, Mux2/3
  Radiator to PHX/1 -> PHX to Freeze Plug/2
  PHX to Freeze Plug/1 -> SALT_Exit_Temp/1
  Demand From Workspace/1 -> Switch/3
  Clock/1 -> Switch/2
  Switch/1 -> Mux2/4
  Constant1/1 -> Switch/1

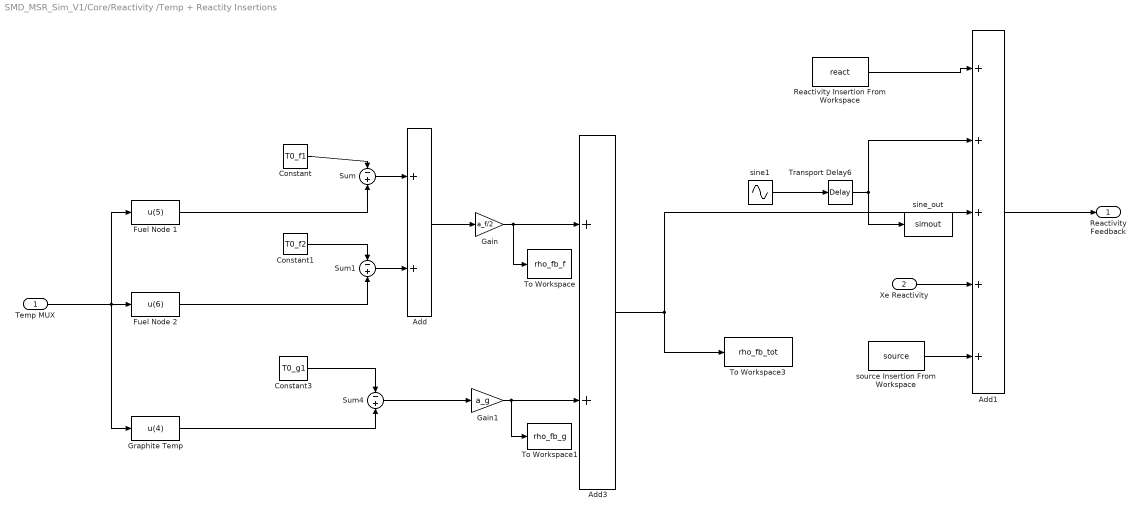
== system SMD_MSR_Sim_V1/Core/Reactivity /Temp + Reactity Insertions ==
  "Temp MUX " : Inport
  Xe Reactivity : Inport  Port=2
  Add : Sum
  Add1 : Sum  Inputs=+++++
  Add3 : Sum
  Constant : Constant  Value=T0_f1
  Constant1 : Constant  Value=T0_f2
  Constant3 : Constant  Value=T0_g1
  "Fuel Node 1 " : Fcn  Expr=u(5)
  Fuel Node 2 : Fcn  Expr=u(6)
  Gain : Gain  Gain=a_f/2
  Gain1 : Gain  Gain=a_g
  Graphite Temp : Fcn  Expr=u(4)
  Reactivity Insertion From Workspace : FromWorkspace  VariableName=react  SampleTime=1  Interpolate=off  OutputAfterFinalValue=Holding final value
  Sum : Sum  Inputs=-|+
  Sum1 : Sum  Inputs=-|+
  Sum4 : Sum  Inputs=-|+
  To Workspace : ToWorkspace  VariableName=rho_fb_f  SampleTime=-1
  To Workspace1 : ToWorkspace  VariableName=rho_fb_g  SampleTime=-1
  To Workspace3 : ToWorkspace  VariableName=rho_fb_tot  SampleTime=-1
  Transport Delay6 : TransportDelay  DelayTime=1000  BufferSize=4096
  sine1 : Sin  Amplitude=sin_mag  Frequency=omega  SampleTime=0
  sine_out : ToWorkspace  VariableName=simout  SampleTime=-1
  source Insertion From Workspace : FromWorkspace  VariableName=source  SampleTime=1  Interpolate=off  OutputAfterFinalValue=Holding final value
  Reactivity Feedback : Outport
  wires:
  Constant3/1 -> Sum4/1
  Sum/1 -> Add/1
  Add1/1 -> Reactivity Feedback/1
  Gain1/1 -> To Workspace1/1, Add3/2
  "Fuel Node 1 "/1 -> Sum/2
  Reactivity Insertion From Workspace/1 -> Add1/1
  Add/1 -> Gain/1
  "Temp MUX "/1 -> "Fuel Node 1 "/1, Graphite Temp/1, Fuel Node 2/1
  Add3/1 -> To Workspace3/1, Add1/3
  Sum1/1 -> Add/2
  Graphite Temp/1 -> Sum4/2
  Constant1/1 -> Sum1/1
  Sum4/1 -> Gain1/1
  Constant/1 -> Sum/1
  Transport Delay6/1 -> sine_out/1, Add1/2
  Gain/1 -> To Workspace/1, Add3/1
  sine1/1 -> Transport Delay6/1
  Fuel Node 2/1 -> Sum1/2
  Xe Reactivity/1 -> Add1/4
  source Insertion From Workspace/1 -> Add1/5

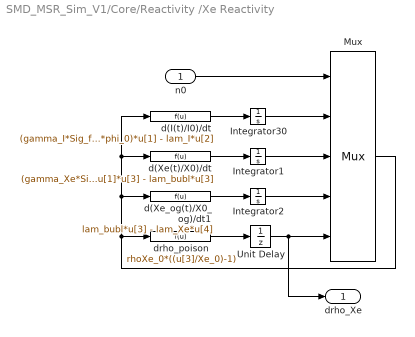
== system SMD_MSR_Sim_V1/Core/Reactivity /Xe Reactivity ==
  n0 : Inport
  Integrator1 : Integrator  InitialCondition=Xe_0
  Integrator2 : Integrator  InitialCondition=Xe_og
  Integrator30 : Integrator  InitialCondition=I_0
  Mux : Mux  Inputs=5
      settings: DisplayOption=signals
  Unit Delay : UnitDelay  SampleTime=-1  HasFrameUpgradeWarning=on
  d(I(t)/I0)/dt : Fcn  Expr=(gamma_I*Sig_f_msdr*phi_0)*u[1] - lam_I*u[2]
  d(Xe(t)/X0)/dt : Fcn  Expr=(gamma_Xe*Sig_f_msdr*phi_0)*u[1] + lam_I*u[2] - lam_Xe*u[3] - sig_Xe*phi_0*u[1]*u[3] - lam_bubl*u[3]
  d(Xe_og(t)/X0_og)/dt1 : Fcn  Expr=lam_bubl*u[3] - lam_Xe*u[4]
  drho_poison : Fcn  Expr=rhoXe_0*((u[3]/Xe_0)-1)
  drho_Xe : Outport
  wires:
  Integrator1/1 -> Mux/3
  Mux/1 -> d(Xe_og(t)/X0_og)/dt1/1, d(I(t)/I0)/dt/1, d(Xe(t)/X0)/dt/1, drho_poison/1
  Integrator2/1 -> Mux/4
  Unit Delay/1 -> Mux/5, drho_Xe/1
  n0/1 -> Mux/1
  drho_poison/1 -> Unit Delay/1
  d(Xe(t)/X0)/dt/1 -> Integrator1/1
  Integrator30/1 -> Mux/2
  d(Xe_og(t)/X0_og)/dt1/1 -> Integrator2/1
  d(I(t)/I0)/dt/1 -> Integrator30/1

== system SMD_MSR_Sim_V1/DHRS /Variant Subsystem/Normal_DHRS ==
  time : Inport
  "Normal_DHRS " : Fcn  Expr=(DHRS_Power-Power_Bleed)/(1+exp(ln(1/Epsilon - 1)*(1 - (u(1)-DHRS_time)/DHRS_TIME_K)))+Power_Bleed
  DHRS : Outport
  wires:
  "Normal_DHRS "/1 -> DHRS/1
  time/1 -> "Normal_DHRS "/1

== matlab function SMD_MSR_Sim_V1/DHRS /Variant Subsystem/Broken_DHRS ==
  data: time input; DHRS output; DHRS_time input; rm_power input; slug_time input
function DHRS = brokenDHRS(time,DHRS_time,rm_power,slug_time)

if (time >= DHRS_time) && (time <= DHRS_time + slug_time)
    DHRS = rm_power;
else 
    DHRS = 0;
end    

% impulse =  t==0;
% unitstep = t>=0;
% ramp = t.*unitstep;
% quad = t.^2.*unitstep;
